simulink model "testJacobianModel1DOF"  (R2022a)
settings: Solver=VariableStepAuto  StartTime=0.0  StopTime=10.0  RelTol=1e-3
undefined symbols (not defined in the file or in its folder): armAttachOffset, smiData, X, Y, Z
libraries: nesl_utility x108, sm_lib x30, robotmaniplib x2
(part 2 of 2)

== matlab function testJacobianModel1DOF/State_Output2/QuatToDCM ==
  data: q input; mat output
function mat  = callQuatToDCM(q)

[mat] = quatToDCM(q);

== matlab function testJacobianModel1DOF/State_Output2/QuatToEuler321 ==
  data: q input; euler output
function euler  = callQuatToEuler321(q)


[euler] = quatToEuler_321(q);

== matlab function testJacobianModel1DOF/State_Output2/formPoseMat ==
  data: rotMat input; mat output; posVec input
function mat  = callFormPoseMat(rotMat,posVec)


[mat] = formPoseMat(rotMat,posVec);

== matlab function testJacobianModel1DOF/State_Output3/MATLAB Function ==
  data: qin input; qout output
function qout = call_quatconj(qin)

qout = zeros(1,4);
qout = quatconj(qin');

== matlab function testJacobianModel1DOF/State_Output3/QuatToDCM ==
  data: q input; mat output
function mat  = callQuatToDCM(q)

[mat] = quatToDCM(q);

== matlab function testJacobianModel1DOF/State_Output3/QuatToEuler321 ==
  data: q input; euler output
function euler  = callQuatToEuler321(q)


[euler] = quatToEuler_321(q);

== matlab function testJacobianModel1DOF/State_Output3/formPoseMat ==
  data: rotMat input; mat output; posVec input
function mat  = callFormPoseMat(rotMat,posVec)


[mat] = formPoseMat(rotMat,posVec);

== matlab function testJacobianModel1DOF/ShoulderAssm_1/State_Output4/MATLAB Function ==
  data: qin input; qout output
function qout = call_quatconj(qin)

qout = zeros(1,4);
qout = quatconj(qin');

== matlab function testJacobianModel1DOF/ShoulderAssm_1/State_Output4/QuatToDCM ==
  data: q input; mat output
function mat  = callQuatToDCM(q)

[mat] = quatToDCM(q);

== matlab function testJacobianModel1DOF/ShoulderAssm_1/State_Output4/QuatToEuler321 ==
  data: q input; euler output
function euler  = callQuatToEuler321(q)


[euler] = quatToEuler_321(q);

== matlab function testJacobianModel1DOF/ShoulderAssm_1/State_Output4/formPoseMat ==
  data: rotMat input; mat output; posVec input
function mat  = callFormPoseMat(rotMat,posVec)


[mat] = formPoseMat(rotMat,posVec);

== matlab function testJacobianModel1DOF/ShoulderAssm_1/State_Output1/MATLAB Function ==
  data: qin input; qout output
function qout = call_quatconj(qin)

qout = zeros(1,4);
qout = quatconj(qin');

== matlab function testJacobianModel1DOF/ShoulderAssm_1/State_Output1/QuatToDCM ==
  data: q input; mat output
function mat  = callQuatToDCM(q)

[mat] = quatToDCM(q);

== matlab function testJacobianModel1DOF/ShoulderAssm_1/State_Output1/QuatToEuler321 ==
  data: q input; euler output
function euler  = callQuatToEuler321(q)


[euler] = quatToEuler_321(q);

== matlab function testJacobianModel1DOF/ShoulderAssm_1/State_Output1/formPoseMat ==
  data: rotMat input; mat output; posVec input
function mat  = callFormPoseMat(rotMat,posVec)


[mat] = formPoseMat(rotMat,posVec);

== matlab function testJacobianModel1DOF/ShoulderAssm_1/State_Output2/MATLAB Function ==
  data: qin input; qout output
function qout = call_quatconj(qin)

qout = zeros(1,4);
qout = quatconj(qin');

== matlab function testJacobianModel1DOF/ShoulderAssm_1/State_Output2/QuatToDCM ==
  data: q input; mat output
function mat  = callQuatToDCM(q)

[mat] = quatToDCM(q);

== matlab function testJacobianModel1DOF/ShoulderAssm_1/State_Output2/QuatToEuler321 ==
  data: q input; euler output
function euler  = callQuatToEuler321(q)


[euler] = quatToEuler_321(q);

== matlab function testJacobianModel1DOF/ShoulderAssm_1/State_Output2/formPoseMat ==
  data: rotMat input; mat output; posVec input
function mat  = callFormPoseMat(rotMat,posVec)


[mat] = formPoseMat(rotMat,posVec);

== matlab function testJacobianModel1DOF/State_Output1/MATLAB Function ==
  data: qin input; qout output
function qout = call_quatconj(qin)

qout = zeros(1,4);
qout = quatconj(qin');

== matlab function testJacobianModel1DOF/State_Output1/QuatToDCM ==
  data: q input; mat output
function mat  = callQuatToDCM(q)

[mat] = quatToDCM(q);
